simulink model "controlWithMeasurementDelay_model"  (R2017a)
settings: Solver=VariableStepAuto  StartTime=0.0  StopTime=simulatietijd  MinStep=1e-3  RelTol=1e-9  EnableMultiTasking=on
values from neighbouring files (symbols this model uses):
  K_p = 10^(-5)*rho*g*R    (= 1.5)    [controlWithMeasurementDelay.m]
  Kc = Kc_help(i)    [PIDTuning.m]    (also in PIDcontroller.m = 5; controlWithMeasurementDelay.m = 2)
  p_na = 3    [controlWithMeasurementDelay.m]
  p_voor = 2    [controlWithMeasurementDelay.m]
  t_step = 5    [PIDcontroller.m]    (also in controlWithMeasurementDelay.m = 1800)
  tau = 1/sys.den(2)    [PIDTuning.m]    (also in controlWithMeasurementDelay.m = 300; margin.m = 300)
  td = 1.5    [PIDTuning.m]    (also in controlWithMeasurementDelay.m = 120)
settings Model: Creator=wrquaghe  LastModifiedBy=geert
settings DataIOCC: LimitDataPoints=on
settings OptimizationCC: LifeSpan=inf
settings DebuggingCC: AllowSymbolicDim=off  SFUnexpectedBacktrackingDiag=warning  SFNoUnconditionalDefaultTransitionDiag=warning  SFExecutionAtInitializationDiag=none
settings ModelReferenceCC: PropagateSignalLabelsOutOfModel=off
settings GRTTargetCC: TargetLangStandard=C89/C90 (ANSI)
settings ConfigComp: CovMetricSettings=dw  CovHtmlReporting=on  CovSaveCumulativeToWorkspaceVar=on  CovSaveSingleToWorkspaceVar=on  CovExternalEMLEnable=off

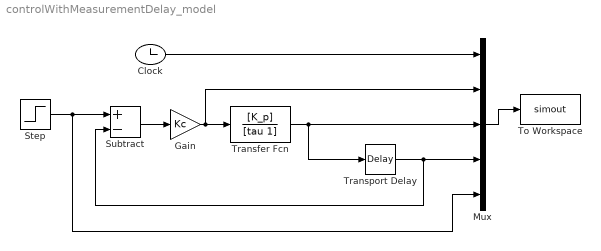
== system controlWithMeasurementDelay_model ==
  Clock : Clock
  Gain : Gain  Gain=Kc
  Mux : Mux  Inputs=5
  Step : Step  Time=t_step  Before=p_voor  After=p_na  SampleTime=0
  Subtract : Sum  Inputs=+-
  To Workspace : ToWorkspace  VariableName=simout  SampleTime=-1
  Transfer Fcn : TransferFcn  Numerator=[K_p]  Denominator=[tau 1]
  Transport Delay : TransportDelay  DelayTime=td
  wires:
  Clock/1 -> Mux/1
  Transfer Fcn/1 -> Transport Delay/1, Mux/3
  Mux/1 -> To Workspace/1
  Transport Delay/1 -> Subtract/2, Mux/4
  Step/1 -> Mux/5, Subtract/1
  Subtract/1 -> Gain/1
  Gain/1 -> Mux/2, Transfer Fcn/1
